simulink model "Cau7"  (R2021b)
settings: Solver=FixedStepAuto  StartTime=0.0  StopTime=inf  RelTol=1e-3
undefined symbols (not defined in the file or in its folder): magnitude
libraries: commchan3 x1, commsink2 x1, commutil2 x1, dspstat3 x1, commrandsrc3 x1, dspsigops x1
settings Model: Creator=ICTLAB  LastModifiedBy=ICTLAB
settings DataIOCC: ReturnWorkspaceOutputs=off

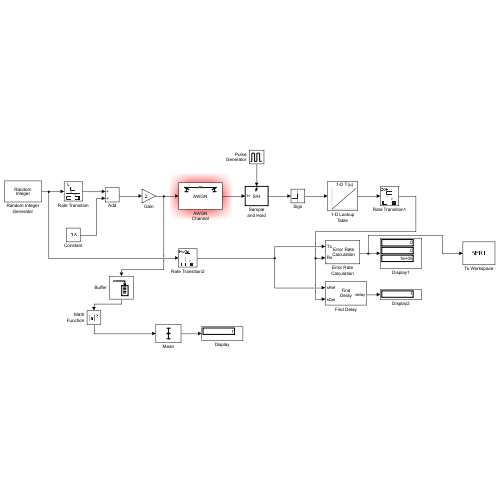
[thumbnail: Simulink's stored preview of the top-level diagram]
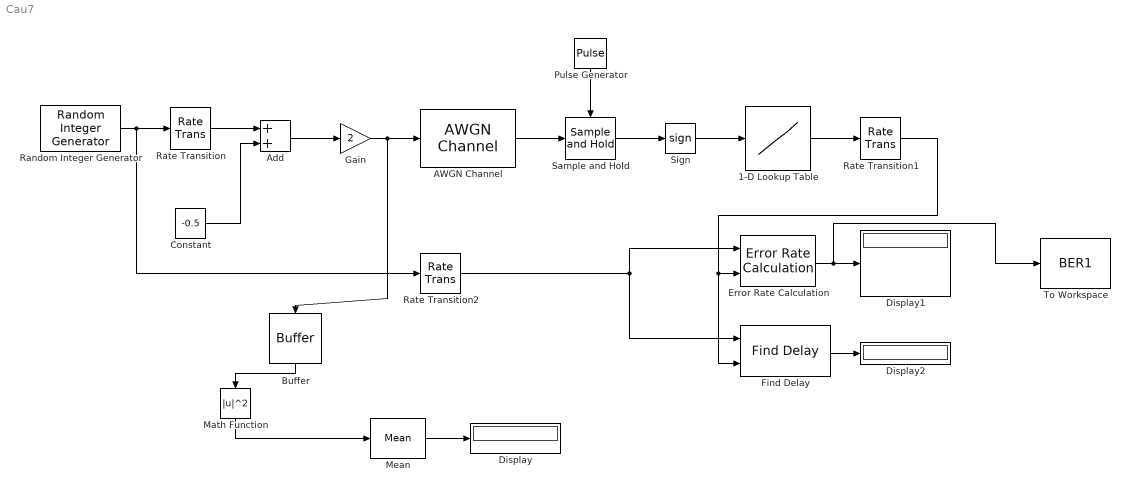
== system Cau7 ==
  1-D Lookup Table : Lookup_n-D  NumberOfTableDimensions=1  BreakpointsForDimension1=[-1 1]  Table=[0 1]  InternalRulePriority=Speed  RndMeth=Simplest  InputSameDT=on
  AWGN Channel : commchan3/AWGN Channel  InputProcessing=Columns as channels (frame based)  seed=67  noiseMode="Signal to noise ratio  (Eb/No)"  EbNodB=EbNo  EsNodB=10  SNRdB=10  bitsPerSym=1  Ps=1  Tsym=1/200000  variance=1
  Add : Sum
  Buffer : Buffer  OutputFrames=off
  Constant : Constant  Value=-0.5
  Display : Display
  Display1 : Display
  Display2 : Display
  Error Rate Calculation : commsink2/Error Rate Calculation  N=1  st_delay=0  cp_mode=Entire frame  subframe=[]  PMode=Port  WsName=ErrorVec  RsMode2=off  stop=on  numErr=1e4  maxBits=1e5
  Find Delay : commutil2/Find Delay  corrLength=200  chgSigOP=off  stopUpdate=off  numConstDelay=3
      settings: SourceProductBaseCode=CM
  Gain : Gain  Gain=2
  Math Function : Math  Operator=magnitude^2  SaturateOnIntegerOverflow=on
  Mean : dspstat3/Mean  run=off  InputProcessing=Columns as channels (frame based)  reset_popup=None  directionMode=Each column  dimension=1  roiEnable=off  roiType=Rectangles  roiPortion=Entire ROI  roiOutput=Individual statistics for each ROI  roiFlag=off  roundingMode=Floor  overflowMode=off  outputDataTypeStr=Inherit: Same as accumulator  outputMin=[]  outputMax=[]  outputLastDataTypeStr=Inherit: Same as accumulator
  Pulse Generator : DiscretePulseGenerator  PulseType=Time based  Period=1/4000  PulseWidth=50
  Random Integer Generator : commrandsrc3/Random Integer Generator  SetSize=2  SeedSource=Auto  Seed=0  SampleTime=1/4000  SamplesPerFrame=1  OutputDataType=double  SimulateUsing=Interpreted execution
  Rate Transition : RateTransition  OutPortSampleTime=1/200000
  Rate Transition1 : RateTransition  OutPortSampleTime=1/4000
  Rate Transition2 : RateTransition  OutPortSampleTime=1/4000
  Sample and Hold : dspsigops/Sample and Hold  trig=Rising edge  initCond=0  latchinput=off
  Sign : Signum
  To Workspace : ToWorkspace  VariableName=BER1  SampleTime=-1
      settings: MaxDataPoints=1
  wires:
  Random Integer Generator/1 -> Rate Transition2/1, Rate Transition/1
  Rate Transition/1 -> Add/1
  Constant/1 -> Add/2
  Add/1 -> Gain/1
  Gain/1 -> Buffer/1, AWGN Channel/1
  AWGN Channel/1 -> Sample and Hold/1
  Pulse Generator/1 -> Sample and Hold/Trigger
  Sample and Hold/1 -> Sign/1
  Sign/1 -> 1-D Lookup Table/1
  1-D Lookup Table/1 -> Rate Transition1/1
  Buffer/1 -> Math Function/1
  Math Function/1 -> Mean/1
  Mean/1 -> Display/1
  Rate Transition2/1 -> Find Delay/1, Error Rate Calculation/1
  Rate Transition1/1 -> Find Delay/2, Error Rate Calculation/2
  Error Rate Calculation/1 -> To Workspace/1, Display1/1
  Find Delay/1 -> Display2/1
